simulink model "ATOM_pred_sim_variable_rear_ratio_lateral"  (R2026a)
settings: Solver=ode4  StopTime=15  FixedStep=0.01
model workspace (MAT data in the model file):
  vehicle : object (value not decoded)
symbols that are objects in the model workspace (value not decoded): vehicle
undefined symbols (not defined in the file or in its folder): delta_f_LUT, gain4WS_LUT, k_ref_LUT, kappa_gain_BP, planning_validator, rr_gain_BP, rr_LUT, stanley, velocity_smoother
(part 4 of 4)

== matlab function ATOM_pred_sim_variable_rear_ratio_lateral/Lateral run()1/CalculateStanley/getData/Calculate Errors/calcYawErrorStanley ==
  data: ego_pose input Bus: KinematicStateBus; yaw_err output; nearest_pose input Bus: PoseBusStanley
function yaw_err = calcYawErrorStanley(ego_pose, nearest_pose)

%% ============================================================
% CALCULATE YAW ERROR
%
% Equivalent to:
%
% Autoware:
%
% data.yaw_err = normalize_radian(
%       tf2::getYaw(current_pose.orientation) -
%       tf2::getYaw(nearest_pose.orientation));
%
% Stanley adaptation:
%
% - current_pose refers to FRONT AXLE
% - nearest_pose is the interpolated reference pose
%   on the reference trajectory
%
% ============================================================


%% Extract yaw

qx = ego_pose.pose.orientation.x;
qy = ego_pose.pose.orientation.y;
qz = ego_pose.pose.orientation.z;
qw = ego_pose.pose.orientation.w;

x = nearest_pose.orientation.x;
y = nearest_pose.orientation.y;
z = nearest_pose.orientation.z;
w = nearest_pose.orientation.w;

current_yaw = QuaternionToYaw(qx,qy,qz,qw);

reference_yaw = QuaternionToYaw(x,y,z,w);



%% Yaw error

yaw_err = reference_yaw - current_yaw;



%% Normalize angle in [-pi, pi]

yaw_err = wrapToPi(yaw_err);


end

== matlab function ATOM_pred_sim_variable_rear_ratio_lateral/Lateral run()1/CalculateStanley/getData/ChooseCurvature ==
  data: curvature_pred input; curvature output; curvature_curr input
function curvature = ChooseCurvature(curvature_pred, curvature_curr)

% =========================================
%
% Left turns: curvature > 0
% Right turns: curvature < 0
%
% =========================================

curvature_max = sin(2*0.7)/(2*cos(-0.7));

if abs(curvature_pred) >= abs(curvature_curr)
    if abs(curvature_pred) >= curvature_max
        sign_k = sign(curvature_pred);
        curvature = sign_k*curvature_max;
    else
        curvature = curvature_pred;
    end
else
    if abs(curvature_curr) >= curvature_max
        sign_k = sign(curvature_curr);
        curvature = sign_k*curvature_max;
    else
        curvature = curvature_curr;
    end


end

== matlab function ATOM_pred_sim_variable_rear_ratio_lateral/Lateral run()1/CalculateStanley/getData/Plot Nearest Pose ==
  settings: updateMethod=DISCRETE
  data: nearest_pose input
function plotNearestPose(nearest_pose)

persistent hFig
persistent ax
persistent hX
persistent hY

persistent X_history
persistent Y_history
persistent time_history

persistent k

%% ============================================================
% Initialization
%% ============================================================

if isempty(k)

    k = 1;

    X_history = nearest_pose.position.x;
    Y_history = nearest_pose.position.x;
    time_history = 0;

    hFig = figure(14);
    clf

    ax = axes(hFig);

    hold(ax,'on')
    grid(ax,'on')

    xlabel(ax,'Sample')
    ylabel(ax,'Error')

    title(ax,'Nearest_pose')

    hX = plot(time_history,...
        X_history,...
        'b','LineWidth',2);

    hY = plot(time_history,...
        Y_history,...
        'r','LineWidth',2);

    legend(ax,...
        {'X nearest','Y nearest'},...
        'Location','best');

else

    k = k + 1;

    time_history(end+1) = k;
    X_history(end+1) = nearest_pose.position.x;
    Y_history(end+1) = nearest_pose.position.y;

    set(hX,...
        'XData',time_history,...
        'YData',X_history);

    set(hY,...
        'XData',time_history,...
        'YData',Y_history);

end

xlim(ax,[0 max(100,k)])

drawnow limitrate

end

== matlab function ATOM_pred_sim_variable_rear_ratio_lateral/Lateral run()1/CalculateStanley/getData/calcNearestPoseInterpStanley ==
  data: self_pose input Bus: KinematicStateBus; trajectory input Bus: TrajectoryDataBus; nearest_pose output Bus: PoseBusStanley; max_dist input; max_yaw input; nearest_idx output
function [nearest_pose,nearest_idx]  = calcNearestPoseInterpStanley( ...
    self_pose, ...
    trajectory, ...
    max_dist, ...
    max_yaw)


%% ============================================================
% CALC NEAREST POSE INTERPOLATION FOR STANLEY CONTROLLER
%
% Equivalent to:
%
% MPCUtils::calcNearestPoseInterp()
%
% Differences with MPC:
%
% - Input trajectory is directly Trajectory message
% - No MPCTrajectory conversion
% - No relative_time prediction
% - Reference is already transformed to FRONT AXLE
%
% The function returns the continuous closest pose of the
% front axle on the reference trajectory.
%
% ============================================================


N = length(trajectory.pose.position.x);



%% ============================================================
% Initialization for code generation
% ============================================================

nearest_pose = struct();

nearest_pose.position.x = 0;
nearest_pose.position.y = 0;
nearest_pose.orientation.x = 0;
nearest_pose.orientation.y = 0;
nearest_pose.orientation.z = 0;
nearest_pose.orientation.w = 0;

nearest_idx = 1;

% nearest_velocity = 0;



if N == 0

    return

end



%% ============================================================
% Step 1:
% Find nearest trajectory index
%
% Equivalent to:
%
% findFirstNearestIndexWithSoftConstraints()
%
% ============================================================


nearest_idx = findFirstNearestIndexWithSoftConstraints( ...
    trajectory,...
    self_pose,...
    max_dist,...
    max_yaw);



%% ============================================================
% Single point trajectory
%
% Equivalent Autoware:
%
% if traj.size()==1
%
% ============================================================


if N == 1

    nearest_pose.x = trajectory.pose.position.x(1);
    nearest_pose.y = trajectory.pose.position.y(1);

    nearest_pose.orientation.x = trajectory.pose.orientation.qx(1);
    nearest_pose.orientation.y = trajectory.pose.orientation.qy(1);
    nearest_pose.orientation.z = trajectory.pose.orientation.qz(1);
    nearest_pose.orientation.w = trajectory.pose.orientation.qw(1);

    % nearest_velocity = trajectory.longitudinal_velocity_mps(1);

    return

end



%% ============================================================
% Step 2:
% Determine interpolation segment
%
% Equivalent to:
%
% calcLongitudinalOffset()
%
% ============================================================


if nearest_idx == 1

    prev_idx = 1;
    next_idx = 2;


elseif nearest_idx == N

    prev_idx = N-1;
    next_idx = N;


else


    p_nearest = [
        trajectory.pose.position.x(nearest_idx)
        trajectory.pose.position.y(nearest_idx)
        ];


    p_next = [
        trajectory.pose.position.x(nearest_idx+1)
        trajectory.pose.position.y(nearest_idx+1)
        ];


    signed_length = calcLongitudinalOffset( ...
        p_nearest,...
        p_next,...
        [self_pose.pose.position.x self_pose.pose.position.y]');


    if signed_length <= 0

        prev_idx = nearest_idx-1;
        next_idx = nearest_idx;

    else

        prev_idx = nearest_idx;
        next_idx = nearest_idx+1;

    end

end



%% ============================================================
% Step 3:
% Linear interpolation
%
% Equivalent to:
%
% nearest_pose.position =
% (1-ratio)*prev + ratio*next
%
% ============================================================


p_prev = [
    trajectory.pose.position.x(prev_idx)
    trajectory.pose.position.y(prev_idx)
];


p_next = [
    trajectory.pose.position.x(next_idx)
    trajectory.pose.position.y(next_idx)
];



segment_length = norm(p_next-p_prev);



% avoid division by zero

if segment_length < 1e-5


    nearest_pose.position.x = trajectory.pose.position.x(nearest_idx);
    nearest_pose.position.y = trajectory.pose.position.y(nearest_idx);


    nearest_pose.orientation.x = trajectory.pose.orientation.qx(nearest_idx);
    nearest_pose.orientation.y = trajectory.pose.orientation.qy(nearest_idx);
    nearest_pose.orientation.z = trajectory.pose.orientation.qz(nearest_idx);
    nearest_pose.orientation.w = trajectory.pose.orientation.qw(nearest_idx);

    % nearest_velocity = trajectory.longitudinal_velocity_mps(nearest_idx);


    return

end



%% Projection of ego on segment

offset = calcLongitudinalOffset( ...
    p_prev,...
    p_next,...
    [self_pose.pose.position.x self_pose.pose.position.y]');


ratio = min(max(offset / segment_length,0),1);



%% Interpolated position

nearest_pose.position.x = ...
    (1-ratio)*p_prev(1)+ratio*p_next(1);


nearest_pose.position.y = ...
    (1-ratio)*p_prev(2)+ratio*p_next(2);



%% ============================================================
% Yaw interpolation
%
% Equivalent:
%
% normalize_radian()
%
% ============================================================


yaw_prev = QuaternionToYaw( ...
    trajectory.pose.orientation.qx(prev_idx),...
    trajectory.pose.orientation.qy(prev_idx),...
    trajectory.pose.orientation.qz(prev_idx),...
    trajectory.pose.orientation.qw(prev_idx));


yaw_next = QuaternionToYaw( ...
    trajectory.pose.orientation.qx(next_idx),...
    trajectory.pose.orientation.qy(next_idx),...
    trajectory.pose.orientation.qz(next_idx),...
    trajectory.pose.orientation.qw(next_idx));


yaw_error = wrapToPi(yaw_prev-yaw_next);


nearest_yaw = wrapToPi( ...
    yaw_next + (1-ratio)*yaw_error);

[qx,qy,qz,qw] = yawToQuaternion(nearest_yaw);

nearest_pose.orientation.x = qx;
nearest_pose.orientation.y = qy;
nearest_pose.orientation.z = qz;
nearest_pose.orientation.w = qw;



% %% ============================================================
% % Velocity interpolation
% %
% % Stanley adaptation:
% %
% % The velocity is used for:
% % - gain scheduling
% % - softening factor
% %
% % ============================================================
% 
% 
% v_prev = trajectory.longitudinal_velocity_mps(prev_idx);
% 
% v_next = trajectory.longitudinal_velocity_mps(next_idx);
% 
% 
% nearest_velocity = ...
%     (1-ratio)*v_prev + ratio*v_next;


end

== matlab function ATOM_pred_sim_variable_rear_ratio_lateral/Lateral run()1/CalculateStanley/getData/calcNearestPoseInterpStanley1 ==
  data: self_pose input Bus: KinematicStateBus; trajectory input Bus: TrajectoryDataBus; nearest_pose output Bus: PoseBusStanley; max_dist input; max_yaw input; nearest_idx output
function [nearest_pose,nearest_idx]  = calcNearestPoseInterpStanley( ...
    self_pose, ...
    trajectory, ...
    max_dist, ...
    max_yaw)


%% ============================================================
% CALC NEAREST POSE INTERPOLATION FOR STANLEY CONTROLLER
%
% Equivalent to:
%
% MPCUtils::calcNearestPoseInterp()
%
% Differences with MPC:
%
% - Input trajectory is directly Trajectory message
% - No MPCTrajectory conversion
% - No relative_time prediction
% - Reference is already transformed to FRONT AXLE
%
% The function returns the continuous closest pose of the
% front axle on the reference trajectory.
%
% ============================================================


N = length(trajectory.pose.position.x);



%% ============================================================
% Initialization for code generation
% ============================================================

nearest_pose = struct();

nearest_pose.position.x = 0;
nearest_pose.position.y = 0;
nearest_pose.orientation.x = 0;
nearest_pose.orientation.y = 0;
nearest_pose.orientation.z = 0;
nearest_pose.orientation.w = 0;

nearest_idx = 1;

% nearest_velocity = 0;



if N == 0

    return

end



%% ============================================================
% Step 1:
% Find nearest trajectory index
%
% Equivalent to:
%
% findFirstNearestIndexWithSoftConstraints()
%
% ============================================================


nearest_idx = findFirstNearestIndexWithSoftConstraints( ...
    trajectory,...
    self_pose,...
    max_dist,...
    max_yaw);



%% ============================================================
% Single point trajectory
%
% Equivalent Autoware:
%
% if traj.size()==1
%
% ============================================================


if N == 1

    nearest_pose.x = trajectory.pose.position.x(1);
    nearest_pose.y = trajectory.pose.position.y(1);

    nearest_pose.orientation.x = trajectory.pose.orientation.qx(1);
    nearest_pose.orientation.y = trajectory.pose.orientation.qy(1);
    nearest_pose.orientation.z = trajectory.pose.orientation.qz(1);
    nearest_pose.orientation.w = trajectory.pose.orientation.qw(1);

    % nearest_velocity = trajectory.longitudinal_velocity_mps(1);

    return

end



%% ============================================================
% Step 2:
% Determine interpolation segment
%
% Equivalent to:
%
% calcLongitudinalOffset()
%
% ============================================================


if nearest_idx == 1

    prev_idx = 1;
    next_idx = 2;


elseif nearest_idx == N

    prev_idx = N-1;
    next_idx = N;


else


    p_nearest = [
        trajectory.pose.position.x(nearest_idx)
        trajectory.pose.position.y(nearest_idx)
        ];


    p_next = [
        trajectory.pose.position.x(nearest_idx+1)
        trajectory.pose.position.y(nearest_idx+1)
        ];


    signed_length = calcLongitudinalOffset( ...
        p_nearest,...
        p_next,...
        [self_pose.pose.position.x self_pose.pose.position.y]');


    if signed_length <= 0

        prev_idx = nearest_idx-1;
        next_idx = nearest_idx;

    else

        prev_idx = nearest_idx;
        next_idx = nearest_idx+1;

    end

end



%% ============================================================
% Step 3:
% Linear interpolation
%
% Equivalent to:
%
% nearest_pose.position =
% (1-ratio)*prev + ratio*next
%
% ============================================================


p_prev = [
    trajectory.pose.position.x(prev_idx)
    trajectory.pose.position.y(prev_idx)
];


p_next = [
    trajectory.pose.position.x(next_idx)
    trajectory.pose.position.y(next_idx)
];



segment_length = norm(p_next-p_prev);



% avoid division by zero

if segment_length < 1e-5


    nearest_pose.position.x = trajectory.pose.position.x(nearest_idx);
    nearest_pose.position.y = trajectory.pose.position.y(nearest_idx);


    nearest_pose.orientation.x = trajectory.pose.orientation.qx(nearest_idx);
    nearest_pose.orientation.y = trajectory.pose.orientation.qy(nearest_idx);
    nearest_pose.orientation.z = trajectory.pose.orientation.qz(nearest_idx);
    nearest_pose.orientation.w = trajectory.pose.orientation.qw(nearest_idx);

    % nearest_velocity = trajectory.longitudinal_velocity_mps(nearest_idx);


    return

end



%% Projection of ego on segment

offset = calcLongitudinalOffset( ...
    p_prev,...
    p_next,...
    [self_pose.pose.position.x self_pose.pose.position.y]');


ratio = min(max(offset / segment_length,0),1);



%% Interpolated position

nearest_pose.position.x = ...
    (1-ratio)*p_prev(1)+ratio*p_next(1);


nearest_pose.position.y = ...
    (1-ratio)*p_prev(2)+ratio*p_next(2);



%% ============================================================
% Yaw interpolation
%
% Equivalent:
%
% normalize_radian()
%
% ============================================================


yaw_prev = QuaternionToYaw( ...
    trajectory.pose.orientation.qx(prev_idx),...
    trajectory.pose.orientation.qy(prev_idx),...
    trajectory.pose.orientation.qz(prev_idx),...
    trajectory.pose.orientation.qw(prev_idx));


yaw_next = QuaternionToYaw( ...
    trajectory.pose.orientation.qx(next_idx),...
    trajectory.pose.orientation.qy(next_idx),...
    trajectory.pose.orientation.qz(next_idx),...
    trajectory.pose.orientation.qw(next_idx));


yaw_error = wrapToPi(yaw_prev-yaw_next);


nearest_yaw = wrapToPi( ...
    yaw_next + (1-ratio)*yaw_error);

[qx,qy,qz,qw] = yawToQuaternion(nearest_yaw);

nearest_pose.orientation.x = qx;
nearest_pose.orientation.y = qy;
nearest_pose.orientation.z = qz;
nearest_pose.orientation.w = qw;



% %% ============================================================
% % Velocity interpolation
% %
% % Stanley adaptation:
% %
% % The velocity is used for:
% % - gain scheduling
% % - softening factor
% %
% % ============================================================
% 
% 
% v_prev = trajectory.longitudinal_velocity_mps(prev_idx);
% 
% v_next = trajectory.longitudinal_velocity_mps(next_idx);
% 
% 
% nearest_velocity = ...
%     (1-ratio)*v_prev + ratio*v_next;


end

== matlab function ATOM_pred_sim_variable_rear_ratio_lateral/Lateral run()1/CalculateStanley/getData/calculate curvature current/CalcTrajectoryCurvature ==
  data: trajectory input Bus: TrajectoryDataBus; curvature output; nearest_idx input; idx_dist input
function curvature = ComputeNearestCurvature( ...
    trajectory,...
    nearest_idx, idx_dist)


%% ============================================================
% COMPUTE NEAREST TRAJECTORY CURVATURE
%
% Equivalent to:
%
% autoware::motion_utils::calcTrajectoryCurvatureFrom3Points()
%
% Difference:
%
% - Autoware computes curvature for the whole trajectory
% - Here only the curvature at nearest_idx is required
%   for Stanley controller
%
% Inputs:
%
% trajectory:
%   Reference trajectory
%
% nearest_idx:
%   Nearest trajectory point index
%
% idx_dist:
%   Distance in samples used for three-point fitting
%
%
% Output:
%
% curvature:
%   Local trajectory curvature [1/m]
%
% ============================================================

N = length(trajectory.pose.position.x);



%% Check trajectory length

if N < 3

    curvature = 0;
    return

end



%% Clamp index

nearest_idx = max(1,min(nearest_idx,N));



%% Select three points
%
% Equivalent to Autoware:
%
% p0 = trajectory[i-idx_dist]
% p1 = trajectory[i]
% p2 = trajectory[i+idx_dist]
%
% ============================================================


idx_prev = nearest_idx - min(idx_dist, nearest_idx-1);

idx_next = nearest_idx + min(idx_dist, N-nearest_idx);



p0 = [
    trajectory.pose.position.x(idx_prev),...
    trajectory.pose.position.y(idx_prev)
];


p1 = [
    trajectory.pose.position.x(nearest_idx),...
    trajectory.pose.position.y(nearest_idx)
];


p2 = [
    trajectory.pose.position.x(idx_next),...
    trajectory.pose.position.y(idx_next)
];



%% Compute curvature

curvature = calc_curvature(p0,p1,p2);


end

== matlab function ATOM_pred_sim_variable_rear_ratio_lateral/Lateral run()1/CalculateStanley/getData/calculate curvature current/ComputeIdxDist ==
  data: points_interval input; idx_dist output; vel_smoother input
function idx_dist = ComputeIdxDist( ...
    points_interval, ...
    vel_smoother)

% ComputeIdxDist
%
% Computes the point offset used for trajectory curvature estimation.
%
% The curvature is evaluated using three trajectory points separated by a
% fixed physical distance. Since the trajectory is sampled with a constant
% spatial interval (points_interval), this function converts the desired
% curvature calculation distance into the corresponding point index offset.
%
% In other words, idx_dist represents the number of trajectory points
% corresponding to the specified curvature calculation distance.
%
% Equivalent to the Autoware implementation:
%
% idx_dist = max(int(curvature_calculation_distance / points_interval), 1);

curvature_calculation_distance = vel_smoother(1);

idx_dist = max( ...
    floor(curvature_calculation_distance / points_interval), ...
    1);

== matlab function ATOM_pred_sim_variable_rear_ratio_lateral/Lateral run()1/CalculateStanley/getData/calculate curvature current/ComputePointsInterval ==
  data: input_points_interval input; vel_smoother input; use_resampling input; points_interval output
function points_interval = computePointsInterval(input_points_interval, ...
    vel_smoother, use_resampling)

% Compute the trajectory points interval used for preprocessing.
%
% If resampling is enabled, a constant spatial interval is imposed.
% Otherwise, the original trajectory point spacing is preserved.

sample_ds = vel_smoother(3,1);

if use_resampling

    points_interval = sample_ds;

else

    points_interval = input_points_interval;

end

end

== matlab function ATOM_pred_sim_variable_rear_ratio_lateral/Demanded trajectory generation: smooth Parabola/Smoothed Parabola trajectory ==
  data: x output double; y output double; z output double; qx output double; qy output double; qz output double; qw output double; longitudinal_velocity_mps output double; lateral_velocity_mps output; acceleration_mps2 output; heading_rate_rps output; front_wheel_angle_rad output; rear_wheel_angle_rad output
function [x,y,z,qx,qy,qz,qw,longitudinal_velocity_mps, lateral_velocity_mps, acceleration_mps2, heading_rate_rps, front_wheel_angle_rad, rear_wheel_angle_rad] ...
            = trajectoryGenerator

N=100;

L=50;
Yend=20;


x=zeros(N,1);
y=zeros(N,1);
z=zeros(N,1);


qx=zeros(N,1);
qy=zeros(N,1);
qz=zeros(N,1);
qw=zeros(N,1);

longitudinal_velocity_mps=zeros(N,1);
lateral_velocity_mps=zeros(N,1);
acceleration_mps2=zeros(N,1);
heading_rate_rps=zeros(N,1);
front_wheel_angle_rad=zeros(N,1);
rear_wheel_angle_rad=zeros(N,1);

for i=1:N

    s=(i-1)/(N-1)*L;

    x(i)=s;

    a=Yend/L^2;

    y(i)=a*s^2;

    yaw=atan(2*a*s);


    qx(i)=0;
    qy(i)=0;
    qz(i)=sin(yaw/2);
    qw(i)=cos(yaw/2);


    longitudinal_velocity_mps(i)=5;

end

== matlab function ATOM_pred_sim_variable_rear_ratio_lateral/Lateral run()1/CalculateStanley/getData/calculate curvature predicted/CalcTrajectoryCurvature ==
  data: trajectory input Bus: TrajectoryDataBus; curvature output; nearest_idx input; idx_dist input
function curvature = ComputeNearestCurvature( ...
    trajectory,...
    nearest_idx, idx_dist)


%% ============================================================
% COMPUTE NEAREST TRAJECTORY CURVATURE
%
% Equivalent to:
%
% autoware::motion_utils::calcTrajectoryCurvatureFrom3Points()
%
% Difference:
%
% - Autoware computes curvature for the whole trajectory
% - Here only the curvature at nearest_idx is required
%   for Stanley controller
%
% Inputs:
%
% trajectory:
%   Reference trajectory
%
% nearest_idx:
%   Nearest trajectory point index
%
% idx_dist:
%   Distance in samples used for three-point fitting
%
%
% Output:
%
% curvature:
%   Local trajectory curvature [1/m]
%
% ============================================================

N = length(trajectory.pose.position.x);



%% Check trajectory length

if N < 3

    curvature = 0;
    return

end



%% Clamp index

nearest_idx = max(1,min(nearest_idx,N));



%% Select three points
%
% Equivalent to Autoware:
%
% p0 = trajectory[i-idx_dist]
% p1 = trajectory[i]
% p2 = trajectory[i+idx_dist]
%
% ============================================================


idx_prev = nearest_idx - min(idx_dist, nearest_idx-1);

idx_next = nearest_idx + min(idx_dist, N-nearest_idx);



p0 = [
    trajectory.pose.position.x(idx_prev),...
    trajectory.pose.position.y(idx_prev)
];


p1 = [
    trajectory.pose.position.x(nearest_idx),...
    trajectory.pose.position.y(nearest_idx)
];


p2 = [
    trajectory.pose.position.x(idx_next),...
    trajectory.pose.position.y(idx_next)
];



%% Compute curvature

curvature = calc_curvature(p0,p1,p2);


end

== matlab function ATOM_pred_sim_variable_rear_ratio_lateral/Lateral run()1/CalculateStanley/getData/calculate curvature predicted/ComputeIdxDist ==
  data: points_interval input; idx_dist output; vel_smoother input
function idx_dist = ComputeIdxDist( ...
    points_interval, ...
    vel_smoother)

% ComputeIdxDist
%
% Computes the point offset used for trajectory curvature estimation.
%
% The curvature is evaluated using three trajectory points separated by a
% fixed physical distance. Since the trajectory is sampled with a constant
% spatial interval (points_interval), this function converts the desired
% curvature calculation distance into the corresponding point index offset.
%
% In other words, idx_dist represents the number of trajectory points
% corresponding to the specified curvature calculation distance.
%
% Equivalent to the Autoware implementation:
%
% idx_dist = max(int(curvature_calculation_distance / points_interval), 1);

curvature_calculation_distance = vel_smoother(1);

idx_dist = max( ...
    floor(curvature_calculation_distance / points_interval), ...
    1);

== matlab function ATOM_pred_sim_variable_rear_ratio_lateral/Lateral run()1/CalculateStanley/getData/calculate curvature predicted/ComputePointsInterval ==
  data: input_points_interval input; vel_smoother input; use_resampling input; points_interval output
function points_interval = computePointsInterval(input_points_interval, ...
    vel_smoother, use_resampling)

% Compute the trajectory points interval used for preprocessing.
%
% If resampling is enabled, a constant spatial interval is imposed.
% Otherwise, the original trajectory point spacing is preserved.

sample_ds = vel_smoother(3,1);

if use_resampling

    points_interval = sample_ds;

else

    points_interval = input_points_interval;

end

end

== matlab function ATOM_pred_sim_variable_rear_ratio_lateral/Lateral run()1/MATLAB Function ==
  data: offset_limit input; enable_offset_removal input; steering_offset input; offset output
function offset = getSteeringOffset(offset_limit, enable_offset_removal, steering_offset)

persistent current_offset
if isempty(current_offset)
    current_offset = 0;
end

if enable_offset_removal
    current_offset = steering_offset;
end

offset = min(max(current_offset, -offset_limit), offset_limit);

== matlab function ATOM_pred_sim_variable_rear_ratio_lateral/Lateral run()1/MATLAB Function1 ==
  data: solved input; previous_status output; reason input; previous_status input; previous_reason input; previous_reason output
function [previous_status, previous_reason] = StanleyStatusManager( ...
    solved,...
    reason,...
    previous_status,...
    previous_reason)

% ATTENTION!!!
% In Autoware, stanley_solved_status (originally mpc_solved_status) 
% is a struct, where equivalently:
% - solved = stanley_solved_status.result
% - reason = stanley_solved_status.reason
%
% StanleyStatusManager here is not implemented since it doesn't change the
% implementation of the controller.

previous_status = solved;
previous_reason = reason;

== matlab function ATOM_pred_sim_variable_rear_ratio_lateral/Lateral run()1/RearToFrontOdometry ==
  data: rear_pose input Bus: KinematicStateBus; front_pose_pred output Bus: KinematicStateBus; wheel_base input; tau_max input; d0 input; k_preview input
function front_pose_pred = RearToFrontOdometryPredictive( ...
    rear_pose,...
    wheel_base,...
    tau_max,...
    d0, k_preview)

%% ============================================================
% Predictive Rear -> Front transformation
%
% Position preview:
%   compensates steering actuator delay
%
% Orientation preview:
%   reduced anticipation for Stanley heading error
%
%% ============================================================


%% Preview times

vx = max(abs(rear_pose.twist.linear.x),0.1);

tau_pos = min(tau_max,d0/vx);

tau_yaw = k_preview*tau_pos;



%% Current rear axle state

x_r = rear_pose.pose.position.x;
y_r = rear_pose.pose.position.y;

qx = rear_pose.pose.orientation.x;
qy = rear_pose.pose.orientation.y;
qz = rear_pose.pose.orientation.z;
qw = rear_pose.pose.orientation.w;

yaw = QuaternionToYaw(qx,qy,qz,qw);



%% Vehicle velocities (body frame)

vx_body = rear_pose.twist.linear.x;
vy_body = rear_pose.twist.linear.y;

yaw_rate = rear_pose.twist.angular.z;



%% Body -> World

vx_world = ...
    vx_body*cos(yaw) - ...
    vy_body*sin(yaw);

vy_world = ...
    vx_body*sin(yaw) + ...
    vy_body*cos(yaw);



%% ============================================================
% Predict rear axle position
%% ============================================================

x_r_pred = x_r + vx_world*tau_pos;

y_r_pred = y_r + vy_world*tau_pos;



%% Orientation previews

yaw_pos  = yaw + yaw_rate*tau_pos;

yaw_ctrl = yaw + yaw_rate*tau_yaw;



%% ============================================================
% Predicted front axle position
%% ============================================================

x_f_pred = ...
    x_r_pred + wheel_base*cos(yaw_pos);

y_f_pred = ...
    y_r_pred + wheel_base*sin(yaw_pos);



%% Output

front_pose_pred = rear_pose;

front_pose_pred.pose.position.x = x_f_pred;
front_pose_pred.pose.position.y = y_f_pred;
front_pose_pred.pose.position.z = rear_pose.pose.position.z;


[qx,qy,qz,qw] = yawToQuaternion(yaw_ctrl);

front_pose_pred.pose.orientation.x = qx;
front_pose_pred.pose.orientation.y = qy;
front_pose_pred.pose.orientation.z = qz;
front_pose_pred.pose.orientation.w = qw;



%% Predicted front axle velocity (body frame)

front_pose_pred.twist.linear.x = vx_body;

front_pose_pred.twist.linear.y = ...
    vy_body + yaw_rate*wheel_base;

front_pose_pred.twist.linear.z = rear_pose.twist.linear.z;

end

== matlab function ATOM_pred_sim_variable_rear_ratio_lateral/Lateral run()1/SetStanleyTrajectory/Resample Trajectory ==
  data: trajectory_in input Bus: TrajectoryDataBus; trajectory_out output Bus: TrajectoryDataBus; resample_interval_dist input; nearest_seg_idx input; ego_offset_to_segment input
function trajectory_out = resampleTrajectoryByDistance( ...
    trajectory_in, ...
    resample_interval_dist, ...
    nearest_seg_idx, ...
    ego_offset_to_segment)


%% ============================================================
% RESAMPLE TRAJECTORY BY ARC LENGTH
%
% Equivalent to:
%
% MPCUtils::resampleMPCTrajectoryByDistance()
%
% Adapted for Stanley controller.
%
% Unlike MPC:
% - no MPCTrajectory conversion
% - no curvature resampling
% - no optimization variables
%
% The trajectory is directly interpolated in arc length.
%
% ATTENTION:
% 
% Resampling is not actuated in Simulink since in/out buses present fixed sizes.
% See NOTE at the end of this function.
%
% =============================================================


% N = length(trajectory_in.pose.position.x);
% 
% 
% if N < 2
% 
%     trajectory_out = trajectory_in;
%     return
% 
% end
% 
% 
% 
% %% ============================================================
% % Compute arc length
% % =============================================================
% 
% x = trajectory_in.pose.position.x;
% y = trajectory_in.pose.position.y;
% 
% 
% arc_length = zeros(N,1);
% 
% 
% for i = 2:N
% 
%     dx = x(i)-x(i-1);
%     dy = y(i)-y(i-1);
% 
%     arc_length(i)= ...
%         arc_length(i-1)+sqrt(dx^2+dy^2);
% 
% end
% 
% 
% 
% if isempty(arc_length)
% 
%     trajectory_out = trajectory_in;
%     return
% 
% end
% 
% 
% 
% %% ============================================================
% % Ego position along trajectory
% %
% % Equivalent to:
% %
% % input_arclength(nearest_seg_idx)
% % + ego_offset_to_segment
% %
% % =============================================================
% 
% 
% ego_s = arc_length(nearest_seg_idx) ...
%         + ego_offset_to_segment;
% 
% 
% ego_s = min(max(ego_s,0),arc_length(end));
% 
% 
% 
% %% ============================================================
% % Generate resampling points
% %
% % Same strategy as Autoware:
% % - backward from ego
% % - forward from ego
% %
% % =============================================================
% 
% 
% output_s = [];
% 
% 
% % backward direction
% 
% s = ego_s;
% 
% while s >= 0
% 
%     output_s = [s output_s]; %#ok<AGROW>
% 
%     s = s - resample_interval_dist;
% 
% end
% 
% 
% 
% % forward direction
% 
% s = ego_s + resample_interval_dist;
% 
% 
% while s < arc_length(end)
% 
%     output_s(end+1)=s; % #ok<AGROW>
% 
%     s = s + resample_interval_dist;
% 
% end
% 
% 
% 
% %% ============================================================
% % Interpolation
% % =============================================================
% 
% 
% x_new = interp1( ...
%     arc_length,...
%     x,...
%     output_s,...
%     'linear');
% 
% 
% 
% y_new = interp1( ...
%     arc_length,...
%     y,...
%     output_s,...
%     'linear');
% 
% 
% 
% z = trajectory_in.pose.position.z;
% 
% z_new = interp1( ...
%     arc_length,...
%     z,...
%     output_s,...
%     'linear');
% 
% 
% 
% %% ============================================================
% % Quaternion / yaw interpolation
% %
% % Stanley works with yaw.
% % Therefore interpolate yaw and rebuild quaternion.
% %
% % =============================================================
% 
% 
% yaw = QuaternionToYaw( ...
%     trajectory_in.pose.orientation.qx,...
%     trajectory_in.pose.orientation.qy,...
%     trajectory_in.pose.orientation.qz,...
%     trajectory_in.pose.orientation.qw);
% 
% 
% 
% % avoid discontinuity
% 
% yaw = unwrap(yaw);
% 
% 
% 
% yaw_new = interp1( ...
%     arc_length,...
%     yaw,...
%     output_s,...
%     'linear');
% 
% 
% 
% %% ============================================================
% % Velocity interpolation
% %
% % Autoware uses linear interpolation
% % =============================================================
% 
% 
% vel_new = interp1( ...
%     arc_length,...
%     trajectory_in.longitudinal_velocity_mps,...
%     output_s,...
%     'linear');
% 
% 
% 
% lat_vel_new = interp1( ...
%     arc_length,...
%     trajectory_in.lateral_velocity_mps,...
%     output_s,...
%     'linear');
% 
% 
% 
% acc_new = interp1( ...
%     arc_length,...
%     trajectory_in.acceleration_mps2,...
%     output_s,...
%     'linear');
% 
% 
% 
% %% ============================================================
% % Build output structure
% % =============================================================
% 
% 
% M = length(output_s);
% 
% 
% trajectory_out.pose.position.x = x_new;
% trajectory_out.pose.position.y = y_new;
% trajectory_out.pose.position.z = z_new;
% 
% 
% 
% [qx,qy,qz,qw] = yawToQuaternion(yaw_new);
% 
% 
% 
% trajectory_out.pose.orientation.qx = qx;
% trajectory_out.pose.orientation.qy = qy;
% trajectory_out.pose.orientation.qz = qz;
% trajectory_out.pose.orientation.qw = qw;
% 
% 
% 
% trajectory_out.longitudinal_velocity_mps = vel_new;
% 
% trajectory_out.lateral_velocity_mps = lat_vel_new;
% 
% trajectory_out.acceleration_mps2 = acc_new;
% 
% 
% 
% % steering values are kept
% 
% trajectory_out.front_wheel_angle_rad = ...
%     interp1( ...
%     arc_length,...
%     trajectory_in.front_wheel_angle_rad,...
%     output_s,...
%     'linear');
% 
% 
% trajectory_out.rear_wheel_angle_rad = ...
%     interp1( ...
%     arc_length,...
%     trajectory_in.rear_wheel_angle_rad,...
%     output_s,...
%     'linear');
% 
% 


%% ============================================================
% NOTE (Simulink Implementation)
%
% The trajectory resampling algorithm reported above is equivalent
% to the implementation adopted by Autoware.
%
% However, the main objective of the present work is the development
% and validation of the 4WS Stanley Controller rather than the
% trajectory preprocessing module.
%
% Since Simulink requires fixed-size bus signals, the resampled
% trajectory is not generated in the simulation model.
%
% The original input trajectory is therefore directly propagated to
% the controller, preserving its fixed dimension and avoiding the
% introduction of variable-length signals.
%
% Consequently, the following assignment overwrites the resampled
% trajectory computed above.
%
% ============================================================

trajectory_out = trajectory_in;

end

== matlab function ATOM_pred_sim_variable_rear_ratio_lateral/Lateral run()1/SetStanleyTrajectory/calcLongOffsetToSegment ==
  data: seg_idx input; ego_pose input; trajectory input Bus: TrajectoryDataBus; ego_offset_to_segment output
function ego_offset_to_segment = calcLongOffsetToSegment(seg_idx, ego_pose, trajectory)

ego_offset_to_segment = calcLongitudinalOffsetToSegment(trajectory, seg_idx, ego_pose);

end

== matlab function ATOM_pred_sim_variable_rear_ratio_lateral/Lateral run()1/SetStanleyTrajectory/findFirstNearestSegmentIndexWithSoftConstraints ==
  data: trajectory input; dist_threshold input; yaw_threshold input; nearest_seg_idx output; pose input
function nearest_seg_idx = findNearestSegmentIndexWithSoftConstraints( ...
    trajectory, dist_threshold, yaw_threshold, pose)


%% Step 1:
% Find nearest point index

nearest_idx = findFirstNearestIndexWithSoftConstraints( ...
    trajectory, ...
    pose, ...
    dist_threshold, ...
    yaw_threshold);


N = length(trajectory.pose.position.x);


%% Step 2:
% Convert point index into segment index

% First point
if nearest_idx == 1

    nearest_seg_idx = 1;
    return

end


% Last point
if nearest_idx == N

    nearest_seg_idx = N-1;
    return

end



%% Step 3:
% Determine whether ego lies before or after nearest point
%
% Equivalent to Autoware:
%
% signed_length =
% calcLongitudinalOffsetToSegment(points,
%                                 nearest_idx,
%                                 pose.position)


signed_length = calcLongitudinalOffsetToSegment( ...
    trajectory,...
    nearest_idx,...
    pose);



%% Step 4:
% Choose segment

if signed_length <= 0

    % ego is before nearest point
    %
    % Autoware:
    % return nearest_idx - 1;

    nearest_seg_idx = nearest_idx - 1;


else

    % ego is after nearest point
    %
    % Autoware:
    % return nearest_idx;

    nearest_seg_idx = nearest_idx;

end


end

== matlab function ATOM_pred_sim_variable_rear_ratio_lateral/Lateral run()1/UpdateSteeringOffset ==
  settings: updateMethod=DISCRETE
  data: steering input; twist input Bus: TwistBus; wheel_base input; update_vel_threshold input; update_steer_threshold input; average_num input; offset_limit input; steering_offset output; veh input
function steering_offset = updateSteeringOffset( ...
    steering,...
    twist,...
    wheel_base,...
    update_vel_threshold,...
    update_steer_threshold,...
    average_num,...
    offset_limit, ...
    veh)


persistent offset_storage
persistent count
persistent current_offset

rear_steering_ratio = veh(29);

if isempty(offset_storage)

    offset_storage = zeros(average_num,1);
    count = 0;
    current_offset = 0;

end


%% Current vehicle state

vx = twist.linear.x;
yaw_rate = twist.angular.z;



%% Check if offset update is allowed

update_offset = ...
    abs(vx) > update_vel_threshold && ...
    abs(steering) < update_steer_threshold;



if update_offset


    %% Estimate steering from vehicle motion

    rear_steering = rear_steering_ratio * steering;

    steer_angle_est = atan( ...
        yaw_rate*wheel_base/vx + tan(rear_steering));



    %% Compute offset

    new_offset = steering - steer_angle_est;



    %% Circular buffer

    count = count + 1;


    if count <= average_num

        offset_storage(count) = new_offset;

    else

        % shift left

        offset_storage(1:end-1)=offset_storage(2:end);

        offset_storage(end)=new_offset;

    end



    %% Compute average

    valid_samples = min(count,average_num);

    current_offset = mean(offset_storage(1:valid_samples));


end



%% Saturation (Autoware getOffset)

steering_offset = min(max(current_offset,...
    -offset_limit),...
    offset_limit);

end

== matlab function ATOM_pred_sim_variable_rear_ratio_lateral/Plot demanded trajectory ==
  data: traj input
function plotTrajectory(traj)

persistent hTraj hArrow


x = traj.pose.position.x;
y = traj.pose.position.y;

yaw = zeros(length(x),1);


for i=1:length(x)

    yaw(i)=2*atan2(...
        traj.pose.orientation.qz(i),...
        traj.pose.orientation.qw(i));

end


if isempty(hTraj)

    figure(2)
    clf
    hold on
    grid on
    axis equal

    hTraj=plot(x,y,'b','LineWidth',2);


    step=5;

    hArrow=quiver(...
        x(1:step:end),...
        y(1:step:end),...
        cos(yaw(1:step:end)),...
        sin(yaw(1:step:end)),...
        0.5,...
        'r');

else

    set(hTraj,...
        'XData',x,...
        'YData',y);

end


drawnow limitrate

end

== matlab function ATOM_pred_sim_variable_rear_ratio_lateral/velocity_smoother_node/ApplySteeringRateLimit - velocity_smoother_node/ApplyPreProcess ==
  data: input input Bus: TrajectoryDataBus; use_resempling input boolean; output output Bus: TrajectoryDataBus; points_interval input double
function output = applyPreProcess(input, use_resempling, points_interval)

% ApplyPreProcess
%
% This function reproduces the first stage of Autoware
% SmootherBase::applyPreProcess().
%
% In Autoware, when resampling is enabled, the input trajectory
% is interpolated with a constant spatial interval.
%
% In this Simulink implementation the resampling stage is omitted
% (use_resempling == false)
% The original trajectory points are directly forwarded to the next block.
%

output = input;

end

== matlab function ATOM_pred_sim_variable_rear_ratio_lateral/velocity_smoother_node/ApplySteeringRateLimit - velocity_smoother_node/Step1: Calculate curvature assuming the trajectory points interval is constant./CalcTrajectoryCurvature ==
  data: trajectory input Bus: TrajectoryDataBus; curvature output; idx_dist input
function curvature = ComputeTrajectoryCurvature( ...
    trajectory, ...
    idx_dist)

% ComputeTrajectoryCurvature
%
% Computes the geometric curvature of a trajectory using a three-point
% circle fitting method.
%
% This function reproduces the behavior of:
%
% autoware_motion_utils::calcTrajectoryCurvatureFrom3Points()
%
% used inside:
%
% autoware_velocity_smoother
%
% In the original Autoware implementation, the curvature computation:
%
%   curvature = calc_curvature(p0,p1,p2)
%
% is protected by a C++ try/catch block. If the circle fitting fails
% (for example due to degenerate geometry), Autoware keeps the previous
% curvature value.
%
% MATLAB/Simulink code generation does not support try/catch constructs.
% Therefore this implementation assumes that calc_curvature() is robust
% and handles degenerate cases internally.
%
% Inputs
% -------
% trajectory : struct
%
%   MATLAB representation of Autoware TrajectoryPoints.
%
%   Autoware source:
%
%   autoware_motion_utils/src/trajectory/conversion.cpp
%
%   converts:
%
%       autoware_planning_msgs::msg::Trajectory
%
%   into:
%
%       std::vector<autoware_planning_msgs::msg::TrajectoryPoint>
%
%   via:
%
    % std::vector<autoware_planning_msgs::msg::TrajectoryPoint> convertToTrajectoryPointArray(
    % const autoware_planning_msgs::msg::Trajectory & trajectory)
    % {
    %     std::vector<autoware_planning_msgs::msg::TrajectoryPoint> output(trajectory.points.size());
    %     std::copy(trajectory.points.begin(), trajectory.points.end(), output.begin());
    %     return output;
    % }
%
%
%
%   Each trajectory point contains:
%
%       geometry_msgs/msg/Point pose.position
%
%   with:
%
%       x, y, z
%
%   MATLAB representation:
%
%       trajectory.pose.position.x
%       trajectory.pose.position.y
%       trajectory.pose.position.z
%
%
% idx_dist : scalar
%
%   Number of trajectory samples used as offset for the three-point
%   curvature estimation.
%
%   In Autoware:
%
%       idx_dist =
%       max(floor(curvature_calculation_distance / points_interval),1)
%
%
% Output
% -------
% curvature : Nx1 vector
%
%   Estimated trajectory curvature [1/m].

num_points = length(trajectory.pose.position.x);


%% Not enough trajectory points

% Autoware:
%
% if (trajectory.size() < 3)
% {
%     return vector filled with zeros;
% }

if num_points < 3
    curvature = zeros(num_points,1);
    return;
end


%% Limit idx_dist according to trajectory size

% Autoware:
%
% max_idx_dist =
% floor((trajectory.size()-1)/2)
%
% idx_dist =
% max(1,min(idx_dist,max_idx_dist))

max_idx_dist = floor((num_points-1)/2);

idx_dist = max(1,min(idx_dist,max_idx_dist));


%% Initialize curvature vector

% Autoware:
%
% std::vector<double> k_arr(trajectory.size(),0.0);

curvature = zeros(num_points,1);


%% Three-point curvature estimation

% Autoware:
%
% for (size_t i = 1; i + 1 < trajectory.size(); i++)

% MATLAB indexing:
%
% i = 2 ... N-1

for i = 2:num_points-1


    % Select the three points:
    %
    % p0 : idx_dist samples before
    % p1 : current trajectory point
    % p2 : idx_dist samples after
    %
    % Equivalent to Autoware:
    %
    % p0 = get_point(
    %       trajectory.at(i - min(idx_dist,i)))
    %
    % p1 = get_point(
    %       trajectory.at(i))
    %
    % p2 = get_point(
    %       trajectory.at(
    %       i + min(idx_dist,size-i-1)))


    idx_prev = i - min(idx_dist,i-1);

    idx_curr = i;

    idx_next = i + min(idx_dist,num_points-i);


    % geometry_msgs/msg/Point:
    %
    % float64 x
    % float64 y
    % float64 z

    p0 = [
        trajectory.pose.position.x(idx_prev), ...
        trajectory.pose.position.y(idx_prev), ...
        trajectory.pose.position.z(idx_prev)
        ];

    p1 = [
        trajectory.pose.position.x(idx_curr), ...
        trajectory.pose.position.y(idx_curr), ...
        trajectory.pose.position.z(idx_curr)
        ];

    p2 = [
        trajectory.pose.position.x(idx_next), ...
        trajectory.pose.position.y(idx_next), ...
        trajectory.pose.position.z(idx_next)
        ];


    %% Compute curvature

    % Autoware:
    %
    % try
    % {
    %     curvature = calc_curvature(p0,p1,p2);
    % }
    %
    % catch(...)
    % {
    %     curvature = previous curvature;
    % }
    %
    % try/catch removed because unsupported by Simulink Coder.

    curvature(i) = calc_curvature(p0,p1,p2);


end


%% Boundary curvature completion

% Autoware:
%
% k_arr.at(0) = k_arr.at(1);
% k_arr.back() = k_arr.at(size-2);

curvature(1) = curvature(2);

curvature(end) = curvature(end-1);


end
